simulink model "testCameraOutput"  (R2016a)
settings: configuration reference "AR_Drone_ConfigSet" (kept outside this file)
undefined symbols (not defined in the file or in its folder): TotalBufferLength
libraries: ARdrone_video_lib x5
settings Model: SimulationMode=external  Creator=sannem  LastModifiedBy=sannem
settings ConfigSetRef: SourceLocation=Base Workspace

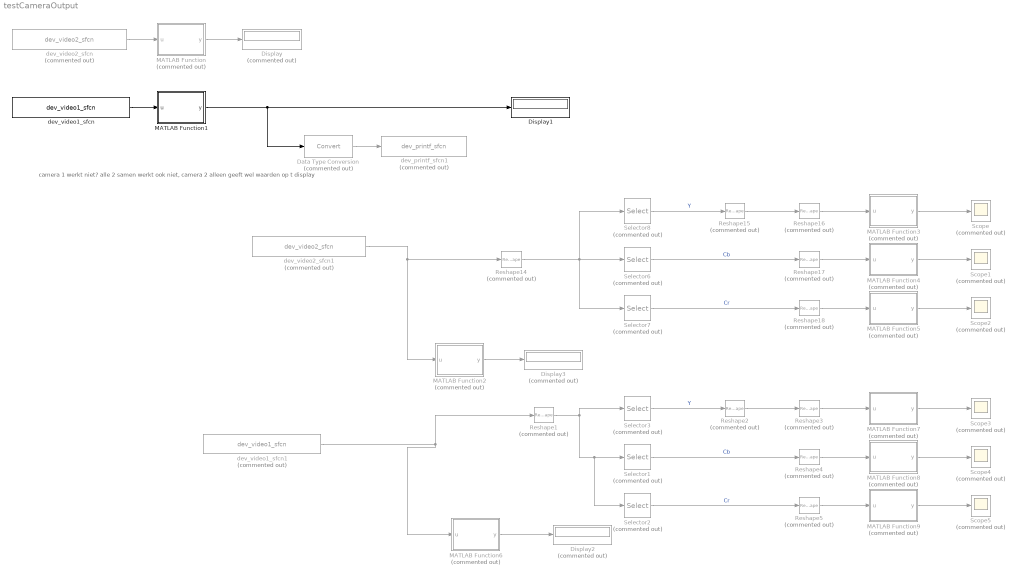
== system testCameraOutput ==
  note: camera 1 werkt niet? alle 2 samen werkt ook niet, camera 2 alleen geeft wel waarden op t display
  Data Type Conversion : DataTypeConversion  Commented=on
  Display : Display  Commented=on
  Display1 : Display
  Display2 : Display  Commented=on
  Display3 : Display  Commented=on
  MATLAB Function : MATLAB Function  Commented=on  TreatAsAtomicUnit=on
  MATLAB Function1 : MATLAB Function  TreatAsAtomicUnit=on
  MATLAB Function2 : MATLAB Function  Commented=on  TreatAsAtomicUnit=on
  MATLAB Function3 : MATLAB Function  Commented=on  TreatAsAtomicUnit=on
  MATLAB Function4 : MATLAB Function  Commented=on  TreatAsAtomicUnit=on
  MATLAB Function5 : MATLAB Function  Commented=on  TreatAsAtomicUnit=on
  MATLAB Function6 : MATLAB Function  Commented=on  TreatAsAtomicUnit=on
  MATLAB Function7 : MATLAB Function  Commented=on  TreatAsAtomicUnit=on
  MATLAB Function8 : MATLAB Function  Commented=on  TreatAsAtomicUnit=on
  MATLAB Function9 : MATLAB Function  Commented=on  TreatAsAtomicUnit=on
  Reshape1 : Reshape  Commented=on  OutputDimensionality=Customize  OutputDimensions=[4 1280*720*2/4]
  Reshape14 : Reshape  Commented=on  OutputDimensionality=Customize  OutputDimensions=[4 320*240*2/4]
  Reshape15 : Reshape  Commented=on  OutputDimensionality=Row vector (2-D)  OutputDimensions=[4 TotalBufferLength/4]
  Reshape16 : Reshape  Commented=on  OutputDimensionality=Customize  OutputDimensions=[320 240]
  Reshape17 : Reshape  Commented=on  OutputDimensionality=Customize  OutputDimensions=[320/2 240]
  Reshape18 : Reshape  Commented=on  OutputDimensionality=Customize  OutputDimensions=[320/2 240]
  Reshape2 : Reshape  Commented=on  OutputDimensionality=Row vector (2-D)  OutputDimensions=[4 TotalBufferLength/4]
  Reshape3 : Reshape  Commented=on  OutputDimensionality=Customize  OutputDimensions=[1280 720]
  Reshape4 : Reshape  Commented=on  OutputDimensionality=Customize  OutputDimensions=[1280/2 720]
  Reshape5 : Reshape  Commented=on  OutputDimensionality=Customize  OutputDimensions=[1280/2 720]
  Scope{,1..5} (6 alike) : Scope  Commented=on
  Selector1 : Selector  Commented=on  NumberOfDimensions=2  InputPortWidth=3  IndexOptions=Index vector (dialog),Index vector (dialog)  Indices=1,[1:460800]  OutputSizes=1,1
  Selector2 : Selector  Commented=on  NumberOfDimensions=2  InputPortWidth=3  IndexOptions=Index vector (dialog),Index vector (dialog)  Indices=3,[1:460800]  OutputSizes=1,1
  Selector3 : Selector  Commented=on  NumberOfDimensions=2  InputPortWidth=3  IndexOptions=Index vector (dialog),Index vector (dialog)  Indices=[2 4],[1:460800]  OutputSizes=1,1
  Selector6 : Selector  Commented=on  NumberOfDimensions=2  InputPortWidth=3  IndexOptions=Index vector (dialog),Index vector (dialog)  Indices=1,[1:38400]  OutputSizes=1,1
  Selector7 : Selector  Commented=on  NumberOfDimensions=2  InputPortWidth=3  IndexOptions=Index vector (dialog),Index vector (dialog)  Indices=3,[1:38400]  OutputSizes=1,1
  Selector8 : Selector  Commented=on  NumberOfDimensions=2  InputPortWidth=3  IndexOptions=Index vector (dialog),Index vector (dialog)  Indices=[2 4],[1:38400]  OutputSizes=1,1
  dev_printf_sfcn1 : ARdrone_video_lib/dev_printf_sfcn  Commented=on  SFunctionSpec=ARpintf_Update(uint8 u1)  SampleTime=-1  ShowSpec=on
  dev_video1_sfcn : ARdrone_video_lib/dev_video1_sfcn  SFunctionSpec=videorabImage1(uint8 y1[1843200])  SampleTime=1/25  ShowSpec=on
  dev_video1_sfcn1 : ARdrone_video_lib/dev_video1_sfcn  Commented=on  SFunctionSpec=videorabImage1(uint8 y1[1843200])  SampleTime=1/10  ShowSpec=on
  dev_video2_sfcn : ARdrone_video_lib/dev_video2_sfcn  Commented=on  SFunctionSpec=videorabImage2(uint8 y1[153600])  SampleTime=1/50  ShowSpec=on
  dev_video2_sfcn1 : ARdrone_video_lib/dev_video2_sfcn  Commented=on  SFunctionSpec=videorabImage2(uint8 y1[153600])  SampleTime=1/25  ShowSpec=on
  wires:
  dev_video2_sfcn/1 -> MATLAB Function/1(u)
  MATLAB Function/1(y) -> Display/1
  dev_video1_sfcn/1 -> MATLAB Function1/1(u)
  MATLAB Function1/1(y) -> Data Type Conversion/1, Display1/1
  MATLAB Function2/1(y) -> Display3/1
  Reshape14/1 -> Selector8/1, Selector7/1, Selector6/1
  Selector6/1 -> Reshape17/1  "Cb"
  Reshape15/1 -> Reshape16/1
  Selector8/1 -> Reshape15/1  "Y"
  Selector7/1 -> Reshape18/1  "Cr"
  Reshape16/1 -> MATLAB Function3/1(u)
  Reshape17/1 -> MATLAB Function4/1(u)
  Reshape18/1 -> MATLAB Function5/1(u)
  MATLAB Function3/1(y) -> Scope/1
  MATLAB Function4/1(y) -> Scope1/1
  MATLAB Function5/1(y) -> Scope2/1
  dev_video2_sfcn1/1 -> Reshape14/1, MATLAB Function2/1(u)
  MATLAB Function6/1(y) -> Display2/1
  Reshape1/1 -> Selector2/1, Selector1/1, Selector3/1
  Selector1/1 -> Reshape4/1  "Cb"
  Reshape2/1 -> Reshape3/1
  Selector3/1 -> Reshape2/1  "Y"
  Selector2/1 -> Reshape5/1  "Cr"
  Reshape3/1 -> MATLAB Function7/1(u)
  Reshape4/1 -> MATLAB Function8/1(u)
  Reshape5/1 -> MATLAB Function9/1(u)
  MATLAB Function7/1(y) -> Scope3/1
  MATLAB Function8/1(y) -> Scope4/1
  MATLAB Function9/1(y) -> Scope5/1
  dev_video1_sfcn1/1 -> MATLAB Function6/1(u), Reshape1/1
  Data Type Conversion/1 -> dev_printf_sfcn1/1

== matlab function testCameraOutput/MATLAB Function1 ==
  data: u input; y output
function y = fcn(u)

y = u(1);

== matlab function testCameraOutput/MATLAB Function ==
  data: u input; y output
function y = fcn(u)

y = mean(u);

== matlab function testCameraOutput/MATLAB Function2 ==
  data: u input; y output
function y = fcn(u)

y = mean(u);

== matlab function testCameraOutput/MATLAB Function3 ==
  data: u input; y output
function y = fcn(u)

y = mean(mean(u));

== matlab function testCameraOutput/MATLAB Function4 ==
  data: u input; y output
function y = fcn(u)

y = mean(mean(u));

== matlab function testCameraOutput/MATLAB Function5 ==
  data: u input; y output
function y = fcn(u)

y = mean(mean(u));

== matlab function testCameraOutput/MATLAB Function6 ==
  data: u input; y output
function y = fcn(u)

y = mean(u);

== matlab function testCameraOutput/MATLAB Function7 ==
  data: u input; y output
function y = fcn(u)

y = u(1,1);

== matlab function testCameraOutput/MATLAB Function8 ==
  data: u input; y output
function y = fcn(u)

y = u(1,1);

== matlab function testCameraOutput/MATLAB Function9 ==
  data: u input; y output
function y = fcn(u)

y = u(1,1);
